simulink model "bramBurst_TransposeMatrix"  (R2021a)
settings: Solver=VariableStepAuto  StartTime=0.0  StopTime=44550  FixedStep=Ts  RelTol=1e-3  EnableMultiTasking=on
InitFcn:
  | model_init_sim;
  | matrix_init;
model workspace (MAT data in the model file):
  mwTaskManagerKernelLatency = 0
  socvcb = containers.Map
  socvcb.serialization.keys = {12.0018310547, 12.001953125, 12.0020751953, 13.0018310547, 13.001953125, 13.0020751953, 14.0018310547, 14.0020751953, 15.0018310547, 15.0020751953, 16.0091552734, 17.0096435547, 30.0006103516, 31.0006103516, 74.0001220703, 74.0092773438, 74.0178222656, 75.0001220703, 75.0092773438, 75.0178222656, 16098.003418, 20393.0119629, 21004.0001221, 22191.0001221}
  socvcb.serialization.values : function handle (value not decoded)
  socvcb.serialization.uniformity = 0
  socvcb.serialization.keyType = 'double'
  socvcb.serialization.valueType = 'any'
undefined symbols (not defined in the file or in its folder): MatrixInput, pAXIDataWidthBytes, pBramAddrWidth, pMaxBankLines, pMaxNumBanks, pNumCols, pNumRows, Ts
libraries: hdlsllib x4, socmemlib x2, simulink x2
settings Model: DataTypeOverride=Off  ExtModeTrigDuration=1  Creator=skuznick  LastModifiedBy=darenlee
settings SolverCC: AlgebraicLoopSolver=TrustRegion  PositivePriorityOrder=on
settings DataIOCC: LimitDataPoints=on  SaveOutput=off  DSMLogging=off  InspectSignalLogs=on  VisualizeSimOutput=off  SaveTime=off
settings OptimizationCC: BlockReduction=off  ConditionallyExecuteInputs=off  DefaultUnderspecifiedDataType=single  EnhancedBackFolding=on  PassReuseOutputArgsAs=Individual arguments  ZeroExternalMemoryAtStartup=off  ZeroInternalMemoryAtStartup=off  EfficientFloat2IntCast=on  MaxStackSize=64  SimCompilerOptimization=on  OptimizeBlockOrder=speed  DifferentSizesBufferReuse=on  OptimizationCustomize=off  EfficientTunableParamExpr=on
settings DebuggingCC: AlgebraicLoopMsg=error  SingleTaskRateTransMsg=error  ParameterPrecisionLossMsg=none  ParameterTunabilityLossMsg=error  FixptConstUnderflowMsg=warning  FixptConstOverflowMsg=warning  AllowSymbolicDim=off  PregeneratedLibrarySubsystemCodeDiagnostic=none  SFUnexpectedBacktrackingDiag=warning  SFNoUnconditionalDefaultTransitionDiag=warning  SFExecutionAtInitializationDiag=none  SFMachineParentedDataDiag=warning  IntegerSaturationMsg=none  ArithmeticOperatorsInVariantConditions=warning
settings HardwareCC: ProdBitPerLong=64  ProdLargestAtomicInteger=LongLong  ProdLargestAtomicFloat=Double  ProdLongLongMode=on  ProdHWDeviceType=ARM Compatible->ARM 64-bit (LP64)  ProdEqTarget=off  HardwareBoardFeatureSet=SoCBlockset
settings SFSimCC: SimUseLocalCustomCode=off  MATLABDynamicMemAlloc=off  CustomCodeUndefinedFunction=UseInterfaceOnly
settings RTWCC: SystemTargetFile=ert.tlc  HardwareBoard=Xilinx Zynq UltraScale+ MPSoC ZCU102 Evaluation Kit  TLCOptions="-aInlineSetEventsForThisBaseRateFcn=TLC_FALSE -aSuppressMultiTaskScheduler=TLC_FALSE  -aRateBasedStepFcn=0"  TemplateMakefile=ert_default_tmf  GenerateReport=on  RTWUseLocalCustomCode=off  Toolchain=Linaro AArch64 Linux v6.3.1  BuildConfiguration=Faster Runs  IncludeHyperlinkInReport=on  LaunchReport=on  GenerateTraceInfo=on  GenerateTraceReport=on  GenerateTraceReportSl=on  GenerateTraceReportSf=on  GenerateTraceReportEml=on
settings CodeAppCC: ForceParamTrailComments=on  IgnoreCustomStorageClasses=off  OperatorAnnotations=on  SimulinkDataObjDesc=on  SFDataObjDesc=on  InsertBlockDesc=on
settings ConfigComp: CovMetricSettings=dw  CovSaveCumulativeToWorkspaceVar=on  CovSaveSingleToWorkspaceVar=on  CovExternalEMLEnable=off  CovSFcnEnable=off

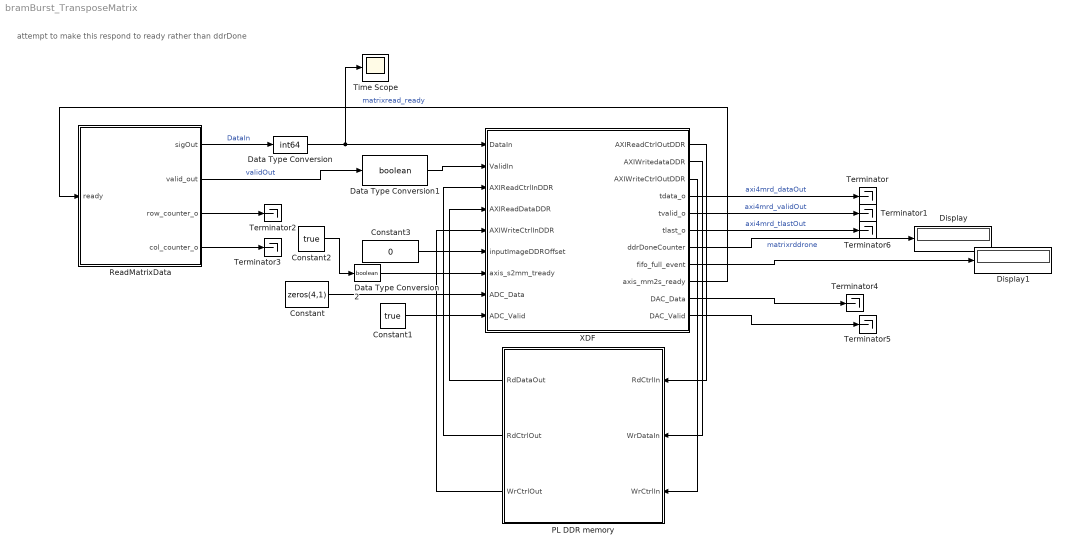
== system bramBurst_TransposeMatrix ==
  note: attempt to make this respond to ready rather than ddrDone
  Constant : Constant  Value=zeros(4,1)  OutDataTypeStr=int16  SampleTime=-1
  Constant1 : Constant  Value=true  OutDataTypeStr=boolean  SampleTime=-1
  Constant2 : Constant  Value=true  SampleTime=-1
  Constant3 : Constant  Value=0  OutDataTypeStr=uint32  SampleTime=-1
  Data Type Conversion : DataTypeConversion  OutDataTypeStr=int64
  Data Type Conversion1 : DataTypeConversion  OutDataTypeStr=boolean
  Data Type Conversion2 : DataTypeConversion  OutDataTypeStr=boolean
  Display : Display
  Display1 : Display
  PL DDR memory : Subsystem
  ReadMatrixData : MATLAB Function  TreatAsAtomicUnit=on  SystemSampleTime=Ts  mask{MatrixInput=MatrixInput, ValidGap=0, GapsInMatrix=40, Ts=Ts}
      mask prompts: MatrixInput "Matrix value"; ValidGap "Valid Gap between columns"; GapsInMatrix "Valid Gap between matrix writes"; Ts "Sample Time"
  Terminator{,1..6} (7 alike) : Terminator
  Time Scope : Scope
  XDF : Subsystem  TreatAsAtomicUnit=on
  wires:
  PL DDR memory/2(RdCtrlOut) -> XDF/3(AXIReadCtrlInDDR)
  PL DDR memory/3(WrCtrlOut) -> XDF/5(AXIWriteCtrlInDDR)
  PL DDR memory/1(RdDataOut) -> XDF/4(AXIReadDataDDR)
  XDF/1(AXIReadCtrlOutDDR) -> PL DDR memory/1(RdCtrlIn)
  XDF/2(AXIWritedataDDR) -> PL DDR memory/2(WrDataIn)
  XDF/3(AXIWriteCtrlOutDDR) -> PL DDR memory/3(WrCtrlIn)
  Constant3/1 -> XDF/6(inputImageDDROffset)
  ReadMatrixData/1(sigOut) -> Data Type Conversion/1  "DataIn"
  ReadMatrixData/2(valid_out) -> Data Type Conversion1/1  "validOut"
  ReadMatrixData/3(row_counter_o) -> Terminator2/1
  ReadMatrixData/4(col_counter_o) -> Terminator3/1
  Data Type Conversion/1 -> Time Scope/1, XDF/1(DataIn)
  XDF/4(tdata_o) -> Terminator/1  "axi4mrd_dataOut"
  XDF/5(tvalid_o) -> Terminator1/1  "axi4mrd_validOut"
  Data Type Conversion1/1 -> XDF/2(ValidIn)
  XDF/8(fifo_full_event) -> Display1/1
  XDF/7(ddrDoneCounter) -> Display/1  "matrixrddrone"
  XDF/9(axis_mm2s_ready) -> ReadMatrixData/1(ready)  "matrixread_ready"
  Constant/1 -> XDF/8(ADC_Data)
  Constant1/1 -> XDF/9(ADC_Valid)
  XDF/10(DAC_Data) -> Terminator4/1
  XDF/11(DAC_Valid) -> Terminator5/1
  Data Type Conversion2/1 -> XDF/7(axis_s2mm_tready)
  XDF/6(tlast_o) -> Terminator6/1  "axi4mrd_tlastOut"
  Constant2/1 -> Data Type Conversion2/1

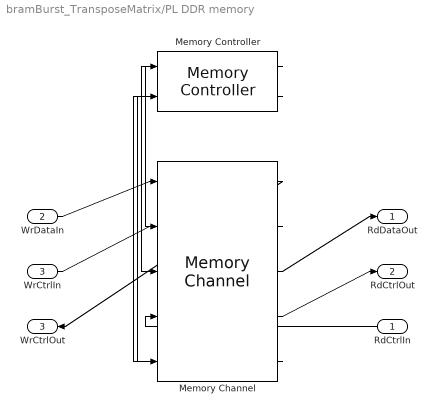
== system bramBurst_TransposeMatrix/PL DDR memory ==
  RdCtrlIn : Inport
  WrDataIn : Inport  Port=2
  WrCtrlIn : Inport  Port=3
  Memory Channel : socmemlib/Memory Channel  InstantiateOnLoad=on  ChannelType=AXI4 Random Access  MRBufferSize=pNumCols*pNumRows*4*4  MRNumBuffers=1  BurstLengthWriterChIf=256  BurstLengthReaderChIf=256  UseValuesFromTargetHardwareResources=off  ReaderWriterUseSameValues=on  FIFODepthWriter=8  FIFODepthReader=8  FIFOAFullDepthWriter=6  FIFOAFullDepthReader=6  ICClockFrequencyWriter=300  ICClockFrequencyReader=300  ICDataWidthWriter=64  ICDataWidthReader=64  ChDimensionsWriterChIf=1  ChTypeWriterChIf=int64  ChFrameSampleTimeWriterChIf=Ts  ChBitPackedWriterChIf=off  OutSigSpecMatchesInSigSpec=on  ChDimensionsReaderChIf=1  ChTypeWithInhReaderChIf=uint8  ChFrameSampleTimeReaderChIf=1  ChBitPackedReaderChIf=off  InsertInactivePixelClocksReaderChIf=off  FrameSizeReaderChIf=160x120p  ProtocolWriter=AXI4  ProtocolReader=AXI4  ChTypeReaderChIf=fixdt(1,64,0)  LastTargetBoard=Xilinx Zynq UltraScale+ MPSoC ZCU102 Evaluation Kit  Beta2Compatible=off  MRRegionSize=62400  DiagnosticLevel=Basic diagnostic signals  MRBaseAddress=hex2dec('00010000')  UseTargetGlobalValues=off  InterruptHandlingTimeWriterChIf=10e-6  BufferEventIDWriterChIf=NOT_USED  BufferLengthReaderChIf=NOT_USED  InterruptHandlingTimeReaderChIf=10e-6  BufferEventIDReaderChIf=NOT_USED
      settings: SourceProductBaseCode=HW
  Memory Controller : socmemlib/Memory Controller  InstantiateOnLoad=on  NumMasters=2  ICArbitrationPolicy=Round robin  UseValuesFromTargetHardwareResources=off  ControllerFrequency=300  ControllerDataWidth=128  BandwidthDerating=2.3  WriteFirstTransferLatency=19  ReadFirstTransferLatency=2  WriteLastTransferLatency=4  ReadLastTransferLatency=1  LastTargetBoard=Xilinx Zynq UltraScale+ MPSoC ZCU102 Evaluation Kit  DiagnosticLevel=Basic diagnostic signals.2  MAX_NUM_MASTERS=12  DDRRefreshLength=4  DDRRefreshInterval=7.8  PlotTimeResolution=100e-6
      settings: SourceProductBaseCode=HW
  RdDataOut : Outport  VectorParamsAs1DForOutWhenUnconnected=off
  RdCtrlOut : Outport  Port=2  VectorParamsAs1DForOutWhenUnconnected=off
  WrCtrlOut : Outport  Port=3  VectorParamsAs1DForOutWhenUnconnected=off
  wires:
  Memory Channel/3 -> RdDataOut/1
  Memory Channel/4 -> RdCtrlOut/1
  Memory Channel/1 -> WrCtrlOut/1
  RdCtrlIn/1 -> Memory Channel/4
  WrDataIn/1 -> Memory Channel/1
  WrCtrlIn/1 -> Memory Channel/2
  Memory Channel/2 -> Memory Controller/1
  Memory Controller/1 -> Memory Channel/3
  Memory Controller/2 -> Memory Channel/5
  Memory Channel/5 -> Memory Controller/2

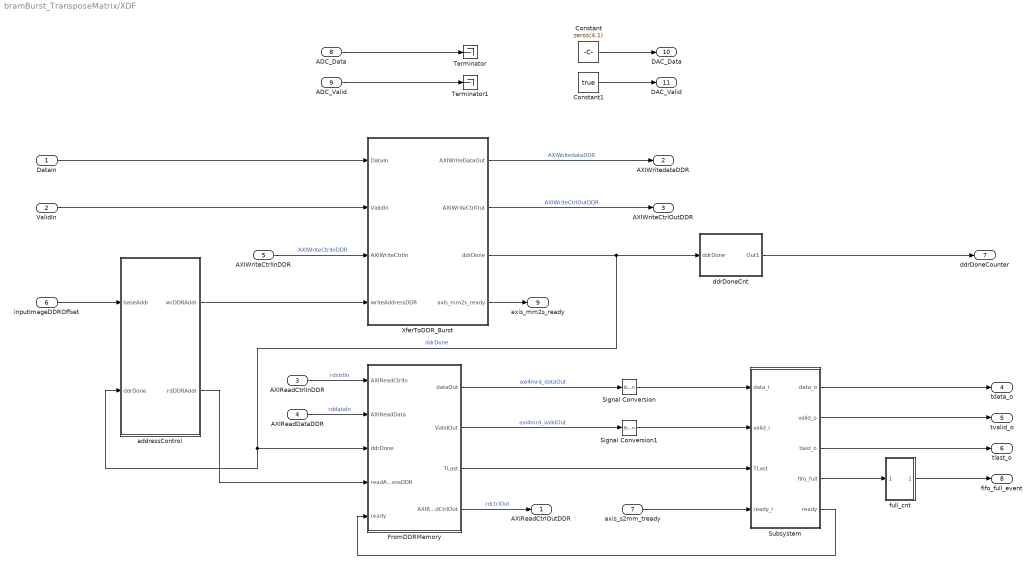
== system bramBurst_TransposeMatrix/XDF ==
  DataIn : Inport
  ValidIn : Inport  Port=2
  AXIReadCtrlInDDR : Inport  Port=3
  AXIReadDataDDR : Inport  Port=4
  AXIWriteCtrlInDDR : Inport  Port=5
  inputImageDDROffset : Inport  Port=6
  axis_s2mm_tready : Inport  Port=7
  ADC_Data : Inport  Port=8
  ADC_Valid : Inport  Port=9
  Constant : Constant  Value=zeros(4,1)  OutDataTypeStr=int16  SampleTime=-1
  Constant1 : Constant  Value=true  OutDataTypeStr=boolean  SampleTime=-1
  FromDDRMemory : Subsystem
  Signal Conversion : SignalConversion  OverrideOpt=off
  Signal Conversion1 : SignalConversion  OverrideOpt=off
  Subsystem : Subsystem
  Terminator : Terminator
  Terminator1 : Terminator
  XferToDDR_Burst : Subsystem  VariantControl=XferToDDR_Burst
  addressControl : Subsystem
  ddrDoneCnt : Subsystem
  full_cnt : Subsystem
  AXIReadCtrlOutDDR : Outport  VectorParamsAs1DForOutWhenUnconnected=off
  AXIWritedataDDR : Outport  Port=2  VectorParamsAs1DForOutWhenUnconnected=off
  AXIWriteCtrlOutDDR : Outport  Port=3  VectorParamsAs1DForOutWhenUnconnected=off
  tdata_o : Outport  Port=4  VectorParamsAs1DForOutWhenUnconnected=off
  tvalid_o : Outport  Port=5
  tlast_o : Outport  Port=6
  ddrDoneCounter : Outport  Port=7
  fifo_full_event : Outport  Port=8
  axis_mm2s_ready : Outport  Port=9
  DAC_Data : Outport  Port=10
  DAC_Valid : Outport  Port=11
  wires:
  AXIWriteCtrlInDDR/1 -> XferToDDR_Burst/3(AXIWriteCtrlIn)  "AXIWriteCtrlInDDR"
  XferToDDR_Burst/1(AXIWriteDataOut) -> AXIWritedataDDR/1  "AXIWritedataDDR"
  XferToDDR_Burst/2(AXIWriteCtrlOut) -> AXIWriteCtrlOutDDR/1  "AXIWriteCtrlOutDDR"
  AXIReadCtrlInDDR/1 -> FromDDRMemory/1(AXIReadCtrlIn)  "rdctrlIn"
  AXIReadDataDDR/1 -> FromDDRMemory/2(AXIReadData)  "rddataIn"
  XferToDDR_Burst/3(ddrDone) -> ddrDoneCnt/1(ddrDone), addressControl/2(ddrDone), FromDDRMemory/3(ddrDone)  "ddrDone"
  FromDDRMemory/1(dataOut) -> Signal Conversion/1  "axi4mrd_dataOut"
  FromDDRMemory/4(AXIReadCtrlOut) -> AXIReadCtrlOutDDR/1  "rdctrlOut"
  DataIn/1 -> XferToDDR_Burst/1(DataIn)
  ValidIn/1 -> XferToDDR_Burst/2(ValidIn)
  FromDDRMemory/2(ValidOut) -> Signal Conversion1/1  "axi4mrd_validOut"
  inputImageDDROffset/1 -> addressControl/1(baseAddr)
  addressControl/1(wrDDRAddr) -> XferToDDR_Burst/4(writeAddressDDR)
  addressControl/2(rdDDRAddr) -> FromDDRMemory/4(readAddressDDR)
  XferToDDR_Burst/4(axis_mm2s_ready) -> axis_mm2s_ready/1
  Signal Conversion/1 -> Subsystem/1(data_i)
  Signal Conversion1/1 -> Subsystem/2(valid_i)
  axis_s2mm_tready/1 -> Subsystem/4(ready_i)
  Subsystem/1(data_o) -> tdata_o/1
  Subsystem/2(valid_o) -> tvalid_o/1
  Subsystem/4(fifo_full) -> full_cnt/1(In1)
  full_cnt/1(Out1) -> fifo_full_event/1
  ddrDoneCnt/1(Out1) -> ddrDoneCounter/1
  Subsystem/5(ready) -> FromDDRMemory/5(ready)
  ADC_Data/1 -> Terminator/1
  ADC_Valid/1 -> Terminator1/1
  Constant/1 -> DAC_Data/1
  Constant1/1 -> DAC_Valid/1
  FromDDRMemory/3(TLast) -> Subsystem/3(TLast)
  Subsystem/3(tlast_o) -> tlast_o/1

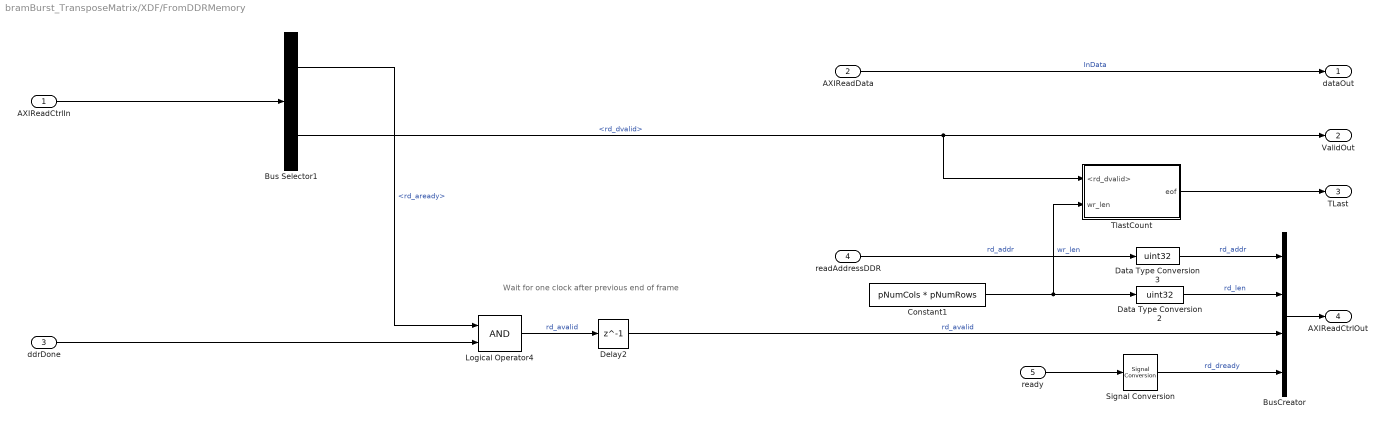
== system bramBurst_TransposeMatrix/XDF/FromDDRMemory ==
  note: Wait for one clock after previous end of frame
  AXIReadCtrlIn : Inport
  AXIReadData : Inport  Port=2
  ddrDone : Inport  Port=3
  readAddressDDR : Inport  Port=4
  ready : Inport  Port=5
  Bus Selector1 : BusSelector  OutputSignals=rd_aready,rd_dvalid
  BusCreator : BusCreator  Inputs=4
  Constant1 : Constant  Value=pNumCols * pNumRows  OutDataTypeStr=uint32  SampleTime=-1
  Data Type Conversion2 : DataTypeConversion  OutDataTypeStr=uint32
  Data Type Conversion3 : DataTypeConversion  OutDataTypeStr=uint32
  Delay2 : Delay  DelayLength=1  InitialCondition=0
  Logical Operator4 : Logic  IconShape=distinctive  AllPortsSameDT=off  OutDataTypeStr=boolean
  Signal Conversion : SignalConversion  OverrideOpt=off
  TlastCount : Subsystem
  dataOut : Outport  VectorParamsAs1DForOutWhenUnconnected=off
  ValidOut : Outport  Port=2
  TLast : Outport  Port=3
  AXIReadCtrlOut : Outport  Port=4  VectorParamsAs1DForOutWhenUnconnected=off
  wires:
  Delay2/1 -> BusCreator/3  "rd_avalid"
  Signal Conversion/1 -> BusCreator/4  "rd_dready"
  Bus Selector1/1 -> Logical Operator4/1  "<rd_aready>"
  BusCreator/1 -> AXIReadCtrlOut/1
  Bus Selector1/2 -> TlastCount/1(<rd_dvalid>), ValidOut/1  "<rd_dvalid>"
  Logical Operator4/1 -> Delay2/1  "rd_avalid"
  AXIReadData/1 -> dataOut/1  "InData"
  Constant1/1 -> TlastCount/2(wr_len), Data Type Conversion2/1  "wr_len"
  Data Type Conversion2/1 -> BusCreator/2  "rd_len"
  AXIReadCtrlIn/1 -> Bus Selector1/1
  Data Type Conversion3/1 -> BusCreator/1  "rd_addr"
  readAddressDDR/1 -> Data Type Conversion3/1  "rd_addr"
  ddrDone/1 -> Logical Operator4/2
  ready/1 -> Signal Conversion/1
  TlastCount/1(eof) -> TLast/1

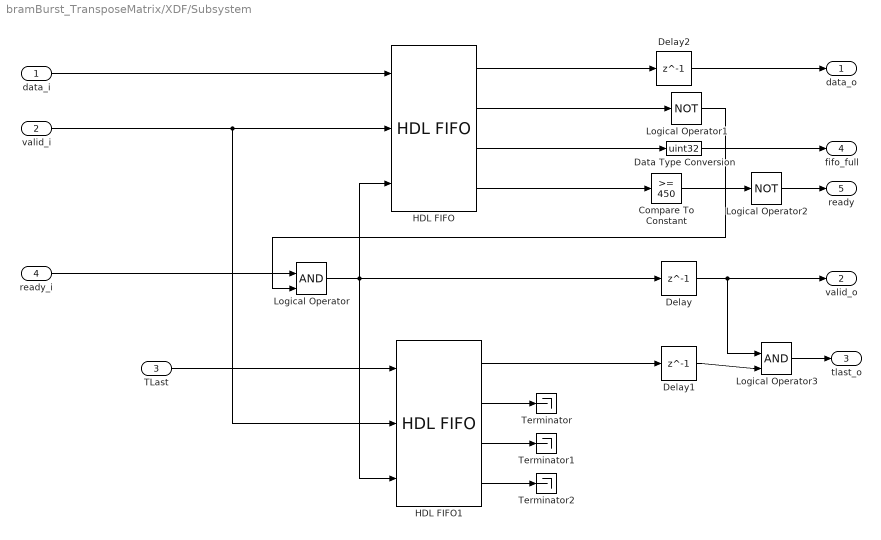
== system bramBurst_TransposeMatrix/XDF/Subsystem ==
  data_i : Inport
  valid_i : Inport  Port=2
  TLast : Inport  Port=3
  ready_i : Inport  Port=4
  Compare To Constant : simulink/Logic and Bit Operations/Compare To Constant  relop=>=  const=450  OutDataTypeStr=boolean
  Data Type Conversion : DataTypeConversion  OutDataTypeStr=uint32
  Delay : Delay  DelayLength=1
  Delay1 : Delay  DelayLength=1
  Delay2 : Delay  DelayLength=1
  HDL FIFO : hdlsllib/HDL RAMs/HDL FIFO  fifo_size=512  mode=FWFT  ratio=1  push_msg=Warning  pop_msg=Warning  show_empty=on  show_full=on  show_num=on  LabelModeActiveChoice_Mode=FWFT
      settings: SourceProductBaseCode=SL
  HDL FIFO1 : hdlsllib/HDL RAMs/HDL FIFO  fifo_size=512  mode=FWFT  ratio=1  push_msg=Warning  pop_msg=Warning  show_empty=on  show_full=on  show_num=on  LabelModeActiveChoice_Mode=FWFT
      settings: SourceProductBaseCode=SL
  Logical Operator : Logic  IconShape=distinctive  AllPortsSameDT=off  OutDataTypeStr=boolean
  Logical Operator1 : Logic  Operator=NOT  IconShape=distinctive  AllPortsSameDT=off  OutDataTypeStr=boolean
  Logical Operator2 : Logic  Operator=NOT  IconShape=distinctive  AllPortsSameDT=off  OutDataTypeStr=boolean
  Logical Operator3 : Logic  IconShape=distinctive  AllPortsSameDT=off  OutDataTypeStr=boolean
  Terminator : Terminator
  Terminator1 : Terminator
  Terminator2 : Terminator
  data_o : Outport
  valid_o : Outport  Port=2
  tlast_o : Outport  Port=3
  fifo_full : Outport  Port=4
  ready : Outport  Port=5
  wires:
  valid_i/1 -> HDL FIFO1/2, HDL FIFO/2
  Logical Operator1/1 -> Logical Operator/2
  HDL FIFO/4 -> Compare To Constant/1
  HDL FIFO/1 -> Delay2/1
  Logical Operator/1 -> HDL FIFO1/3, Delay/1, HDL FIFO/3
  HDL FIFO/3 -> Data Type Conversion/1
  Delay2/1 -> data_o/1
  HDL FIFO/2 -> Logical Operator1/1
  data_i/1 -> HDL FIFO/1
  Data Type Conversion/1 -> fifo_full/1
  ready_i/1 -> Logical Operator/1
  Delay/1 -> Logical Operator3/1, valid_o/1
  Compare To Constant/1 -> Logical Operator2/1
  Logical Operator2/1 -> ready/1
  TLast/1 -> HDL FIFO1/1
  HDL FIFO1/2 -> Terminator/1
  HDL FIFO1/3 -> Terminator1/1
  HDL FIFO1/4 -> Terminator2/1
  Delay1/1 -> Logical Operator3/2
  HDL FIFO1/1 -> Delay1/1
  Logical Operator3/1 -> tlast_o/1

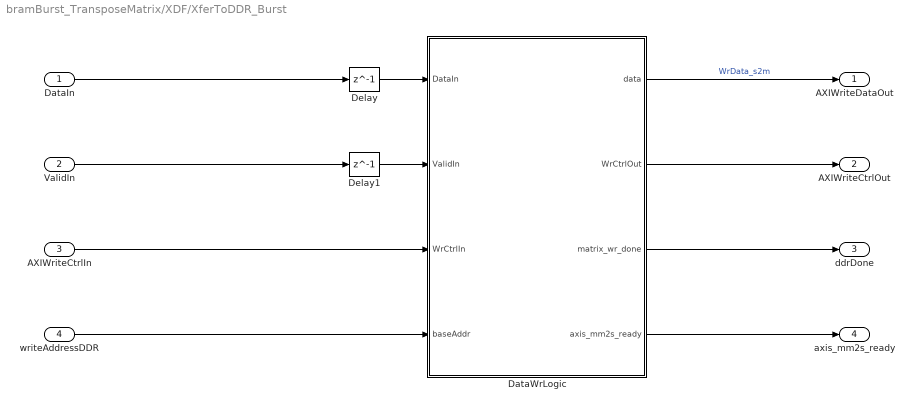
== system bramBurst_TransposeMatrix/XDF/XferToDDR_Burst ==
  DataIn : Inport
  ValidIn : Inport  Port=2
  AXIWriteCtrlIn : Inport  Port=3
  writeAddressDDR : Inport  Port=4
  DataWrLogic : Subsystem
  Delay : Delay  DelayLength=1
  Delay1 : Delay  DelayLength=1
  AXIWriteDataOut : Outport
  AXIWriteCtrlOut : Outport  Port=2
  ddrDone : Outport  Port=3
  axis_mm2s_ready : Outport  Port=4
  wires:
  Delay1/1 -> DataWrLogic/2(ValidIn)
  Delay/1 -> DataWrLogic/1(DataIn)
  DataWrLogic/1(data) -> AXIWriteDataOut/1  "WrData_s2m"
  DataIn/1 -> Delay/1
  DataWrLogic/2(WrCtrlOut) -> AXIWriteCtrlOut/1
  AXIWriteCtrlIn/1 -> DataWrLogic/3(WrCtrlIn)
  DataWrLogic/3(matrix_wr_done) -> ddrDone/1
  ValidIn/1 -> Delay1/1
  writeAddressDDR/1 -> DataWrLogic/4(baseAddr)
  DataWrLogic/4(axis_mm2s_ready) -> axis_mm2s_ready/1

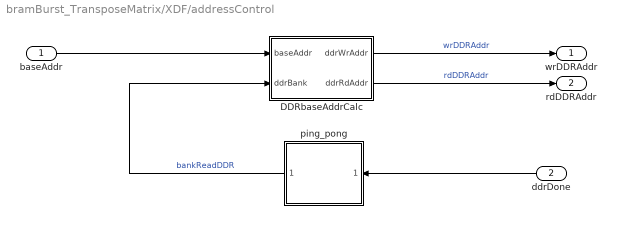
== system bramBurst_TransposeMatrix/XDF/addressControl ==
  baseAddr : Inport
  ddrDone : Inport  Port=2
  DDRbaseAddrCalc : Subsystem
  ping_pong : Subsystem
  wrDDRAddr : Outport
  rdDDRAddr : Outport  Port=2
  wires:
  ping_pong/1(ddrBank) -> DDRbaseAddrCalc/2(ddrBank)  "bankReadDDR"
  ddrDone/1 -> ping_pong/1(ddrDone)
  baseAddr/1 -> DDRbaseAddrCalc/1(baseAddr)
  DDRbaseAddrCalc/1(ddrWrAddr) -> wrDDRAddr/1  "wrDDRAddr"
  DDRbaseAddrCalc/2(ddrRdAddr) -> rdDDRAddr/1  "rdDDRAddr"

== system bramBurst_TransposeMatrix/XDF/ddrDoneCnt ==
  ddrDone : Inport
  Add : Sum  AccumDataTypeStr=uint32
  Data Type Conversion : DataTypeConversion  OutDataTypeStr=int32
  Delay1 : Delay  DelayLength=1
  Out1 : Outport
  wires:
  ddrDone/1 -> Data Type Conversion/1
  Delay1/1 -> Out1/1, Add/2
  Add/1 -> Delay1/1
  Data Type Conversion/1 -> Add/1

== system bramBurst_TransposeMatrix/XDF/full_cnt ==
  In1 : Inport
  Add : Sum  AccumDataTypeStr=uint32
  Delay1 : Delay  DelayLength=1
  Out1 : Outport
  wires:
  In1/1 -> Add/1
  Delay1/1 -> Out1/1, Add/2
  Add/1 -> Delay1/1

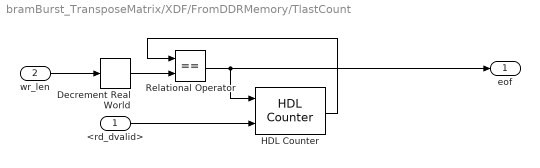
== system bramBurst_TransposeMatrix/XDF/FromDDRMemory/TlastCount ==
  <rd_dvalid> : Inport
  wr_len : Inport  Port=2
  Decrement Real World : simulink/Additional Math & Discrete/Additional Math: Increment - Decrement/Decrement Real World
      settings: SourceProductBaseCode=SL
  HDL Counter : hdlsllib/Sources/HDL Counter  CountType=Free running  CountInit=0  CountStep=1  CountMax=25  CountFromType=Initial value  CountFrom=0  CountResetPort=on  CountLoadPort=off  CountEnbPort=on  CountDirPort=off  CountHitOutputPort=off  CountDataType=Unsigned  CountWordLen=32  CountFracLen=0  CountSampTime=1
  Relational Operator : RelationalOperator  Operator===  OutDataTypeStr=boolean  RndMeth=Simplest
  eof : Outport
  wires:
  wr_len/1 -> Decrement Real World/1
  <rd_dvalid>/1 -> HDL Counter/2
  HDL Counter/1 -> Relational Operator/1
  Relational Operator/1 -> HDL Counter/1, eof/1
  Decrement Real World/1 -> Relational Operator/2

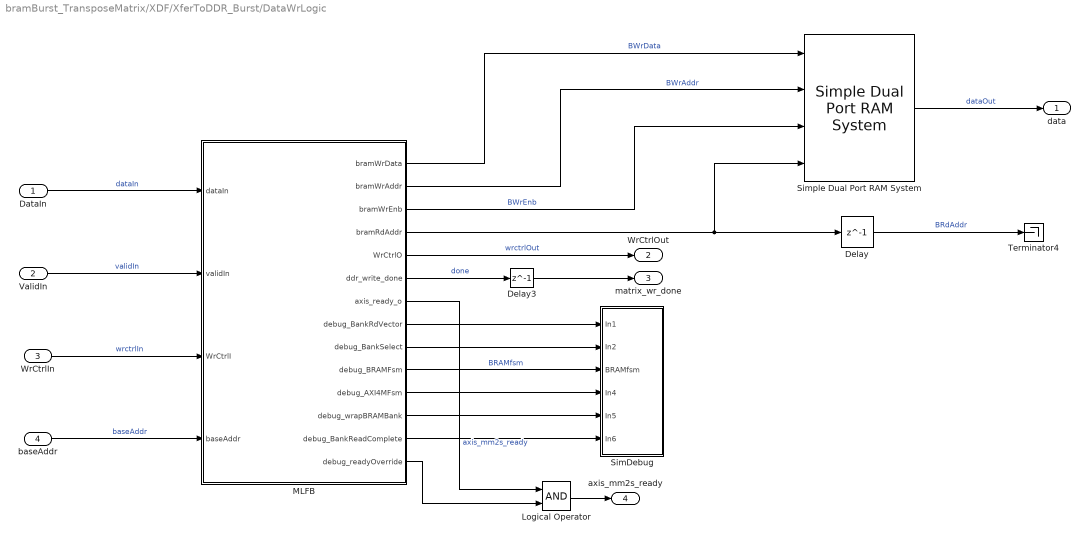
== system bramBurst_TransposeMatrix/XDF/XferToDDR_Burst/DataWrLogic ==
  DataIn : Inport
  ValidIn : Inport  Port=2
  WrCtrlIn : Inport  Port=3
  baseAddr : Inport  Port=4
  Delay : Delay  DelayLength=1
  Delay3 : Delay  DelayLength=1
  Logical Operator : Logic  AllPortsSameDT=off  OutDataTypeStr=boolean
  MLFB : MATLAB Function  TreatAsAtomicUnit=on
  SimDebug : Subsystem
  Simple Dual Port RAM System : hdlsllib/HDL RAMs/Simple Dual Port RAM System  RAMType=Simple dual port  WriteOutputValue=New data  RAMInitialValue=0  SimulateUsing=Code generation
      settings: SourceProductBaseCode=SL
  Terminator4 : Terminator
  data : Outport
  WrCtrlOut : Outport  Port=2
  matrix_wr_done : Outport  Port=3
  axis_mm2s_ready : Outport  Port=4
  wires:
  MLFB/6(ddr_write_done) -> Delay3/1  "done"
  MLFB/5(WrCtrlO) -> WrCtrlOut/1  "wrctrlOut"
  Simple Dual Port RAM System/1 -> data/1  "dataOut"
  baseAddr/1 -> MLFB/4(baseAddr)  "baseAddr"
  WrCtrlIn/1 -> MLFB/3(WrCtrlI)  "wrctrlIn"
  MLFB/1(bramWrData) -> Simple Dual Port RAM System/1  "BWrData"
  ValidIn/1 -> MLFB/2(validIn)  "validIn"
  DataIn/1 -> MLFB/1(dataIn)  "dataIn"
  MLFB/4(bramRdAddr) -> Simple Dual Port RAM System/4, Delay/1
  MLFB/2(bramWrAddr) -> Simple Dual Port RAM System/2  "BWrAddr"
  MLFB/3(bramWrEnb) -> Simple Dual Port RAM System/3  "BWrEnb"
  Delay3/1 -> matrix_wr_done/1
  Delay/1 -> Terminator4/1  "BRdAddr"
  MLFB/7(axis_ready_o) -> Logical Operator/1  "axis_mm2s_ready"
  MLFB/14(debug_readyOverride) -> Logical Operator/2
  Logical Operator/1 -> axis_mm2s_ready/1
  MLFB/8(debug_BankRdVector) -> SimDebug/1(In1)
  MLFB/9(debug_BankSelect) -> SimDebug/2(In2)
  MLFB/10(debug_BRAMFsm) -> SimDebug/3(BRAMfsm)  "BRAMfsm"
  MLFB/11(debug_AXI4MFsm) -> SimDebug/4(In4)
  MLFB/12(debug_wrapBRAMBank) -> SimDebug/5(In5)
  MLFB/13(debug_BankReadComplete) -> SimDebug/6(In6)

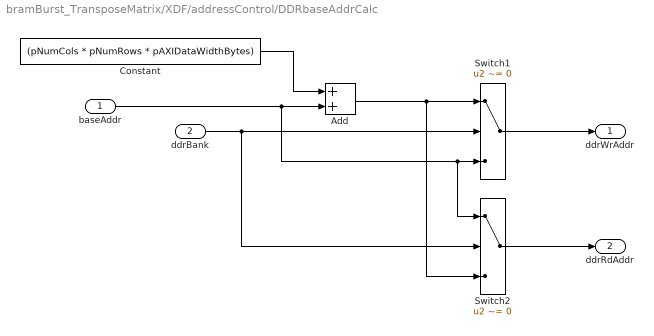
== system bramBurst_TransposeMatrix/XDF/addressControl/DDRbaseAddrCalc ==
  baseAddr : Inport
  ddrBank : Inport  Port=2
  Add : Sum  OutDataTypeStr=uint32
  Constant : Constant  Value=(pNumCols * pNumRows * pAXIDataWidthBytes)  OutDataTypeStr=uint32  SampleTime=-1
  Switch1 : Switch  Criteria=u2 ~= 0
  Switch2 : Switch  Criteria=u2 ~= 0
  ddrWrAddr : Outport
  ddrRdAddr : Outport  Port=2
  wires:
  Constant/1 -> Add/1
  Add/1 -> Switch2/3, Switch1/1
  Switch1/1 -> ddrWrAddr/1
  ddrBank/1 -> Switch2/2, Switch1/2
  baseAddr/1 -> Switch2/1, Switch1/3, Add/2
  Switch2/1 -> ddrRdAddr/1

== system bramBurst_TransposeMatrix/XDF/addressControl/ping_pong ==
  note: if 0 is selected then use first bank (starting at address 0) to read from
      | if 1 is selected then use the second bank (starting at offset) to read from
  ddrDone : Inport
  Logical Operator9 : Logic  Operator=XOR  IconShape=distinctive  AllPortsSameDT=off  OutDataTypeStr=boolean
  Unit Delay1 : UnitDelay  SampleTime=-1  HasFrameUpgradeWarning=on
  sr_latch : Subsystem
  ddrBank : Outport  VectorParamsAs1DForOutWhenUnconnected=off
  wires:
  Unit Delay1/1 -> Logical Operator9/1
  Logical Operator9/1 -> sr_latch/1(S)
  ddrDone/1 -> sr_latch/2(R), Logical Operator9/2
  sr_latch/1(Q) -> Unit Delay1/1, ddrBank/1  "DDR_BankSelect"

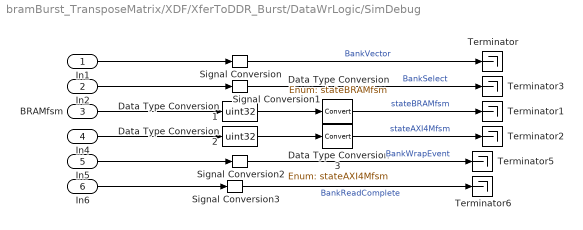
== system bramBurst_TransposeMatrix/XDF/XferToDDR_Burst/DataWrLogic/SimDebug ==
  In1 : Inport
  In2 : Inport  Port=2
  BRAMfsm : Inport  Port=3
  In4 : Inport  Port=4
  In5 : Inport  Port=5
  In6 : Inport  Port=6
  Data Type Conversion : DataTypeConversion  OutDataTypeStr=Enum: stateBRAMfsm
  Data Type Conversion1 : DataTypeConversion  OutDataTypeStr=uint32
  Data Type Conversion2 : DataTypeConversion  OutDataTypeStr=uint32
  Data Type Conversion3 : DataTypeConversion  OutDataTypeStr=Enum: stateAXI4Mfsm
  Signal Conversion{,1..3} (4 alike) : SignalConversion  OverrideOpt=off
  Terminator{,1..3,5..6} (6 alike) : Terminator
  wires:
  Signal Conversion/1 -> Terminator/1  "BankVector"
  Data Type Conversion2/1 -> Data Type Conversion3/1
  Data Type Conversion3/1 -> Terminator2/1  "stateAXI4Mfsm"
  Signal Conversion2/1 -> Terminator5/1  "BankWrapEvent"
  Data Type Conversion1/1 -> Data Type Conversion/1
  Signal Conversion3/1 -> Terminator6/1  "BankReadComplete"
  Signal Conversion1/1 -> Terminator3/1  "BankSelect"
  Data Type Conversion/1 -> Terminator1/1  "stateBRAMfsm"
  BRAMfsm/1 -> Data Type Conversion1/1
  In4/1 -> Data Type Conversion2/1
  In1/1 -> Signal Conversion/1
  In5/1 -> Signal Conversion2/1
  In6/1 -> Signal Conversion3/1
  In2/1 -> Signal Conversion1/1

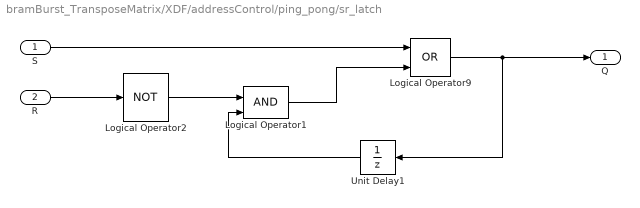
== system bramBurst_TransposeMatrix/XDF/addressControl/ping_pong/sr_latch ==
  S : Inport
  R : Inport  Port=2
  Logical Operator1 : Logic  IconShape=distinctive  AllPortsSameDT=off  OutDataTypeStr=boolean
  Logical Operator2 : Logic  Operator=NOT  IconShape=distinctive  AllPortsSameDT=off  OutDataTypeStr=boolean
  Logical Operator9 : Logic  Operator=OR  IconShape=distinctive  AllPortsSameDT=off  OutDataTypeStr=boolean
  Unit Delay1 : UnitDelay  SampleTime=-1  HasFrameUpgradeWarning=on
  Q : Outport  VectorParamsAs1DForOutWhenUnconnected=off
  wires:
  Logical Operator9/1 -> Q/1, Unit Delay1/1
  Unit Delay1/1 -> Logical Operator1/2
  S/1 -> Logical Operator9/1
  R/1 -> Logical Operator2/1
  Logical Operator2/1 -> Logical Operator1/1
  Logical Operator1/1 -> Logical Operator9/2

== matlab function bramBurst_TransposeMatrix/XDF/XferToDDR_Burst/DataWrLogic/MLFB ==
  data: bramWrData output; bramWrAddr output; bramWrEnb output; bramRdAddr output; WrCtrlO output Bus: WriteControlM2SBusObj; ddr_write_done output; axis_ready_o output; dataIn input; validIn input; WrCtrlI input; baseAddr input; debug_BankRdVector output; debug_BankSelect output; debug_BRAMFsm output; pNumCols parameter; pNumRows parameter; pMaxBankLines parameter; pMaxNumBanks parameter; pAXIDataWidthBytes parameter; debug_AXI4MFsm output; debug_wrapBRAMBank output; debug_BankReadComplete output; pBramAddrWidth parameter; debug_readyOverride output
function [bramWrData, bramWrAddr, bramWrEnb, bramRdAddr, WrCtrlO, ddr_write_done, axis_ready_o, debug_BankRdVector,...
          debug_BankSelect, debug_BRAMFsm, debug_AXI4MFsm, debug_wrapBRAMBank, debug_BankReadComplete, debug_readyOverride] =  ...
burstTranspose(dataIn, validIn, WrCtrlI, baseAddr, pNumCols, pNumRows, pMaxBankLines, pMaxNumBanks, pAXIDataWidthBytes, pBramAddrWidth)

% define FSM States
IDLE = fi(0,0,4,0);
% States for managing the writing to BRAM
LINEBUFFER = fi(1,0,4,0);
LINESTART = fi(3,0,4,0);
% States for managing the writing to DDR
BURSTSTART = fi(1,0,4,0);
BURSTNEXT  = fi(3,0,4,0);
WAITBURSTCOMPLETE = fi(4,0,4,0);
WAITBURSTREADY = fi(5,0,4,0);
WAITONBANKRDY =fi(2,0,4,0);

persistent stateBRAMfsm burstState WrBank RdBank WrData BankRdy...
           WrAddr RdAddr WrEnb colCnt rowCnt WrBankLine RdBankLine...
           WrDone aximWrAddr aximWrValid startRdAddr burstCount...
           aximWrLen aximNumRowsWritten bankWrWrap...
           aximm2s_ready ready_override
           
 
if isempty(stateBRAMfsm)
    stateBRAMfsm = IDLE;
    burstState = IDLE;
    bankWrWrap = false;
    WrBank = fi(0,0,8,0);
    RdBank = fi(0,0,8,0);
    BankRdy = zeros(uint32(pMaxNumBanks),1,'logical');
    WrBankLine = uint16(0);
    RdBankLine = uint16(0);
    WrEnb = false;
    WrDone = false;
    aximWrAddr = uint32(0);
    aximWrLen = uint32(pMaxBankLines);
    aximWrValid = false;
    WrData = cast(0,'like', dataIn);
%     WrAddr = fi(0,0,14,0);
%     RdAddr = fi(0,0,14,0);
    WrAddr = fi(0,0,pBramAddrWidth,0);
    RdAddr = cast(0,'like',WrAddr);
    startRdAddr = cast(0,'like',WrAddr);
    burstCount = uint16(0);
    colCnt = fi(0,0,ceil(log2(pNumCols)),0);
    rowCnt = fi(0,0,ceil(log2(pNumRows)),0);
    aximNumRowsWritten = uint32(0);
    
    % additional ready signals
    aximm2s_ready = true;
    ready_override = true;
end


%% Assign outputs
bramWrData = WrData;
bramWrEnb = WrEnb;
bramWrAddr = WrAddr;
bramRdAddr = RdAddr;
wr_ddr_addr = uint32((aximWrAddr * pAXIDataWidthBytes) + baseAddr);
WrCtrlO = struct('wr_addr', wr_ddr_addr, 'wr_len', aximWrLen, 'wr_valid', aximWrValid);
ddr_write_done = WrDone;
WrDone = false;  % Note: WrDone true for one clock only


%% Ready conditions for axi4-stream
% if there is not enough banks available, check to see if all three are
if ~aximm2s_ready  && (bitconcat(fi(BankRdy,0,1,0)) == 0)
    aximm2s_ready = true;
end

% if ready_override == false
% aximm2s_ready = aximm2s_ready & ready_override;
% end

% if <condition that we are still reading> && (bitconcat(fi(BankRdy,0,1,0)) == 0)
%     aximm2s_ready = true;
% end


%% For debug outputs only
debug_BankRdVector = BankRdy; % display status of each BRAM bank. if a 1 is written to a bank, it means it  has data that has NOT been fully read out yet
debug_BankSelect = WrBank;  % which BRAM bank is selected to write new data to. Zero indexed
debug_wrapBRAMBank = bankWrWrap; % Will occur when we wrap to the first BRAM Bank
debug_BankReadComplete = (RdBankLine == 0); % finished reading a bank (got to end of column) and reset to zero event

debug_BRAMFsm = stateBRAMfsm; % BRAM write state machine
debug_AXI4MFsm = burstState;  % BRAM Read -> DDR4 state machine




%%

% process col and row counts
if WrEnb  % write to BRAM
%     fprintf("+BRAM: %08x @ %u Col %u Row %u WrBankLine %u WrBank %u\n", uint32(WrData), uint32(WrAddr), uint16(colCnt), uint16(rowCnt), WrBankLine, uint16(WrBank));
    if colCnt == pNumCols-1
        if rowCnt == pNumRows-1 % end of matrix
            BankRdy(WrBank+1) = true;
            WrBank(:) = WrBank + 1;
            if WrBank == pMaxNumBanks
                WrBank(:) = 0;
                WrAddr(:) = 0;
            end
            stateBRAMfsm = IDLE;
           
        else
            colCnt(:) = 0;
            rowCnt(:) = rowCnt + 1;
            WrBankLine(:) = WrBankLine + 1;
            if WrBankLine == pMaxBankLines
                BankRdy(WrBank+1) = true;
                if burstState == IDLE
                    burstState = BURSTSTART;
                    startRdAddr(:) = 0;
                end
                WrBankLine(:) = 0;
                WrBank(:) = WrBank + 1;
                % NOTE wrap around to bank 0 
                % The Number of banks might need to change to keep up with
                % the write to DDR rate - keep track of possible collision
                if WrBank == pMaxNumBanks
                    bankWrWrap = true;
                    WrBank(:) = 0;
                    WrAddr(:) = 0;
                end
                if  BankRdy(WrBank+1) == true
                   aximm2s_ready = false;
%                 else
%                    aximm2s_ready = true; 
%                     error('Bank Overrun! Increase number of available banks in BRAM.');
                end
            end
        end
    else
        colCnt(:) = colCnt + 1;
        
        if (colCnt == pNumCols-1) && (rowCnt == pNumRows-1)
             ready_override = false; % dont accept any more data until we are done
        end
    end
end

% reset these after every write
WrEnb = false;

% FSM to manage writing input data to BRAM
switch stateBRAMfsm
    case IDLE
        % first validIn could be on a later clock or on this clock
        if validIn
            WrAddr(:) = 0;
            colCnt(:) = 0;
            rowCnt(:) = 0;
            WrBank(:) = 0;
            BankRdy = zeros(uint32(pMaxNumBanks),1,'logical');
            WrBankLine(:) = 0;
            RdBank(:) = 0;
            
            WrData = dataIn;
            WrEnb = true;
            stateBRAMfsm = LINEBUFFER;
        end
    case LINESTART
        if validIn
            WrData = dataIn;
            WrEnb = true; 
            stateBRAMfsm = LINEBUFFER;
        end
    case LINEBUFFER
        if validIn
            if bankWrWrap
                WrAddr(:) = 0;
                bankWrWrap = false;
            else
                WrAddr(:) = WrAddr + 1;
            end
            WrData = dataIn;
            WrEnb = true; 
        end
end

% FSM To manage the Write to DDR in Bursts in maxBufLines
switch burstState
    case IDLE
    case BURSTSTART
        aximWrAddr(:) = 0; % (bank-1) * maxBufLines;
        RdAddr = startRdAddr ;
        burstCount(:) = 0;
        if BankRdy(RdBank+1) == true
            burstState = WAITBURSTREADY;
        else
            burstState = WAITONBANKRDY;
        end
    case WAITBURSTREADY
        if WrCtrlI.wr_ready
            aximWrValid = true;
            RdAddr(:) = RdAddr + pNumCols;
            burstState(:) = BURSTNEXT;
            burstCount(:) = burstCount + 1;
            if burstCount == aximWrLen
                burstState = WAITBURSTCOMPLETE;
                burstCount(:) = 0;
            end
        else
           aximWrValid = false;
        end
    case BURSTNEXT
        if WrCtrlI.wr_ready
            aximWrValid = true;
            RdAddr(:) = RdAddr + pNumCols;
            burstCount(:) = burstCount + 1;
            if burstCount == aximWrLen
                burstState = WAITBURSTCOMPLETE;
                burstCount(:) = 0;
            end
        else
            aximWrValid = false;
            burstState = WAITBURSTREADY;
        end
    case WAITBURSTCOMPLETE
        aximWrValid = false;
%         if WrCtrlI.wr_complete
        if WrCtrlI.wr_ready  % support pipelined writes (R2020a+)
            aximWrAddr(:) = aximWrAddr + pNumRows;
            % go to next burst of maxBufLines
            startRdAddr(:) = startRdAddr + 1; 
            burstState = WAITBURSTREADY;
            RdBankLine(:) = RdBankLine + 1;
            if RdBankLine == pNumCols   % Reached the end of a bank, need to move to next bank
                RdBankLine(:) = 0;
                BankRdy(RdBank+1) = false;
                RdBank(:) = RdBank + 1;
                if RdBank == pMaxNumBanks
                    RdBank(:) = 0;
                    startRdAddr(:) = 0;
                end
                startRdAddr(:) = uint16(RdBank) * coder.const((pNumCols * pMaxBankLines));  
                aximNumRowsWritten(:) = aximNumRowsWritten + aximWrLen;
                if (pNumRows - aximNumRowsWritten) < pMaxBankLines
                    aximWrLen(:) = pNumRows - aximNumRowsWritten;
                end
                aximWrAddr(:) = aximNumRowsWritten;
                if BankRdy(RdBank+1) == false
                    burstState = WAITONBANKRDY;
%                     fprintf('WAITING for Ready Bank: %u\n', uint32(RdBank));
                end
                if aximNumRowsWritten == pNumRows
                    aximWrLen = uint32(pMaxBankLines);
                    aximNumRowsWritten(:)  = 0;
                    burstState(:) = IDLE;
                    WrDone = true;
                    ready_override = true; % accept new data into BRAM now
                end
            end
            RdAddr(:) = startRdAddr; 
        end        
    case WAITONBANKRDY
        if BankRdy(RdBank+1) == true
            burstState = WAITBURSTREADY;
        end
end


axis_ready_o = aximm2s_ready ;
debug_readyOverride = ready_override;

== matlab function bramBurst_TransposeMatrix/ReadMatrixData ==
  data: sigOut output; valid_out output; MatrixInput parameter; row_counter_o output; col_counter_o output; ValidGap parameter; ready input; GapsInMatrix parameter
function [sigOut,valid_out,row_counter_o,col_counter_o] = fcn(MatrixInput,ValidGap, ready, GapsInMatrix)
    persistent row_counter col_counter stop_write numMatrixWrites gapCounter;
%     ValidGap = 10;
    if isempty(row_counter)
        row_counter = uint32(1);
        col_counter = uint32(1);
        stop_write = false;
        numMatrixWrites = uint32(0);
        gapCounter = uint32(0);
      
    end
    [n_rows,m_cols] = size(MatrixInput);
    max_row_count = n_rows + ValidGap;

    %% Read value from matrix
    if row_counter <= n_rows && ~stop_write && ready
        sigOut = MatrixInput(row_counter,col_counter);
        valid_out = true;
    else
        sigOut = 0; % insert valid gap 
        valid_out = false;
    end
    
    row_counter_o = row_counter;
    col_counter_o = col_counter;
    
    %% Update counters
    if ready
        if row_counter < max_row_count 
            row_counter(:) = row_counter + 1; 
        else          
            
            if col_counter < m_cols
                row_counter(:) = 1;
                col_counter(:) = col_counter + 1; % next column
            else
%                 if gapCounter < GapsInMatrix                    
%                     gapCounter(:) = gapCounter + 1;
%                     valid_out = false;
%                 else
%                   
%                 end
            
                row_counter(:) = 1;
                col_counter(:) = 1; % reset to beginning of matrix

                if numMatrixWrites < inf
                    stop_write = false; % set to true to stop indefinite reads
                else
                    stop_write = true;
                end
                numMatrixWrites  = numMatrixWrites  + 1;             
            end
        end
    else
        valid_out = false;
    end

end
